simulink model "GUI_Model"  (R2026a)
settings: Solver=VariableStepDiscrete  StopTime=100
settings Model: DataDictionary=Architecture_DD.sldd  Creator=jaime  LastModifiedBy=jaime

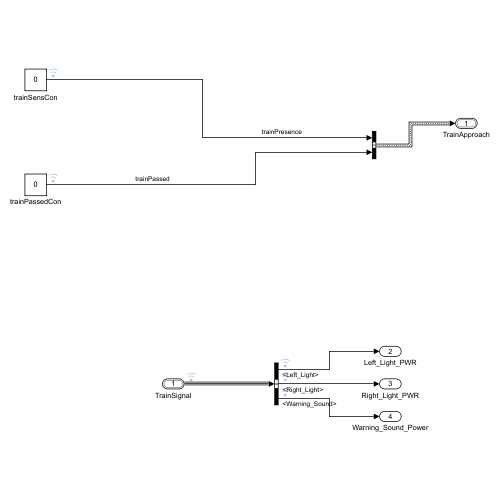
[thumbnail: Simulink's stored preview of the top-level diagram]
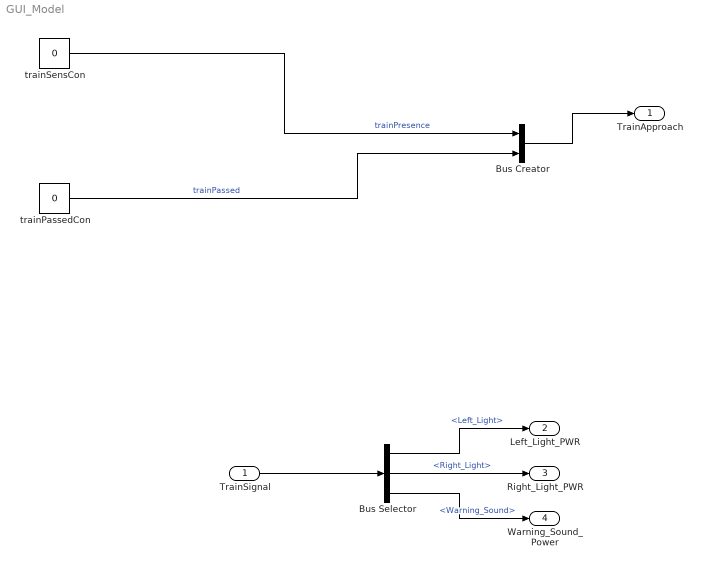
== system GUI_Model ==
  TrainSignal : Inport  OutDataTypeStr=Bus: Node_TrainSigBus
  Bus Creator : BusCreator  Inputs=2  OutDataTypeStr=Bus: Node_TrainSensBus  NonVirtualBus=on
      settings: InheritFromInputs=off
  Bus Selector : BusSelector  OutputSignals=Left_Light,Right_Light,Warning_Sound
  trainPassedCon : Constant  Value=0  OutDataTypeStr=boolean
  trainSensCon : Constant  Value=0  OutDataTypeStr=boolean
  TrainApproach : Outport  OutDataTypeStr=Bus: Node_TrainSensBus
  Left_Light_PWR : Outport  Port=2
  Right_Light_PWR : Outport  Port=3
  Warning_Sound_Power : Outport  Port=4
  wires:
  Bus Creator/1 -> TrainApproach/1
  trainSensCon/1 -> Bus Creator/1  "trainPresence"
  trainPassedCon/1 -> Bus Creator/2  "trainPassed"
  Bus Selector/1 -> Left_Light_PWR/1  "<Left_Light>"
  Bus Selector/2 -> Right_Light_PWR/1  "<Right_Light>"
  Bus Selector/3 -> Warning_Sound_Power/1  "<Warning_Sound>"
  TrainSignal/1 -> Bus Selector/1
